simulink model "ex6"  (R2015a)
settings: Solver=ode3  StartTime=0.0  StopTime=10.0  FixedStep=0.001  RelTol=1e-3
undefined symbols (not defined in the file): g, l
libraries: simulink x1
settings Model: Creator=fschalle  LastModifiedBy=fschalle

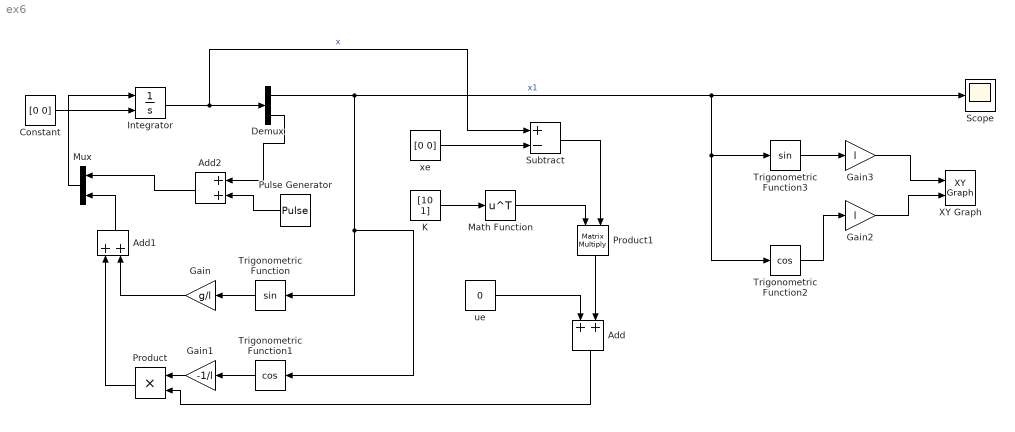
== system ex6 ==
  Add : Sum
  Add1 : Sum
  Add2 : Sum
  Constant : Constant  Value=[0 0]
  Demux : Demux  Outputs=2
  Gain : Gain  Gain=g/l
  Gain1 : Gain  Gain=-1/l
  Gain2 : Gain  Gain=l
  Gain3 : Gain  Gain=l
  Integrator : Integrator  InitialConditionSource=external
  "K " : Constant  Value=[10 1]
  Math Function : Math  Operator=transpose  SaturateOnIntegerOverflow=on
  Mux : Mux  Inputs=2
  Product : Product
  Product1 : Product  Multiplication=Matrix(*)
  Pulse Generator : DiscretePulseGenerator  PulseType=Time based  Amplitude=5  Period=1  PulseWidth=2
  Scope : Scope
      settings: YMin=-7  YMax=7
  Subtract : Sum  Inputs=+-
  Trigonometric Function : Trigonometry
  Trigonometric Function1 : Trigonometry  Operator=cos
  Trigonometric Function2 : Trigonometry  Operator=cos
  Trigonometric Function3 : Trigonometry
  XY Graph : simulink/Sinks/XY Graph  xmin=-1  xmax=1  ymin=-1  ymax=1  st=-1
  ue : Constant  Value=0
  xe : Constant  Value=[0 0]
  wires:
  Constant/1 -> Integrator/2
  Integrator/1 -> Subtract/1, Demux/1  "x"
  Mux/1 -> Integrator/1
  Trigonometric Function/1 -> Gain/1
  Demux/1 -> Trigonometric Function2/1, Trigonometric Function3/1, Scope/1, Trigonometric Function1/1, Trigonometric Function/1  "x1"
  Add1/1 -> Mux/2
  Gain/1 -> Add1/2
  xe/1 -> Subtract/2
  Trigonometric Function1/1 -> Gain1/1
  Gain1/1 -> Product/1
  Product/1 -> Add1/1
  ue/1 -> Add/1
  Add/1 -> Product/2
  Trigonometric Function2/1 -> Gain2/1
  Trigonometric Function3/1 -> Gain3/1
  Gain2/1 -> XY Graph/2
  Gain3/1 -> XY Graph/1
  Product1/1 -> Add/2
  Subtract/1 -> Product1/2
  "K "/1 -> Math Function/1
  Math Function/1 -> Product1/1
  Add2/1 -> Mux/1
  Pulse Generator/1 -> Add2/2
  Demux/2 -> Add2/1
